simulink model "IK_corrado_old"  (R2023a)
settings: Solver=VariableStepAuto  StartTime=0.0  StopTime=15  MaxStep=0.05  RelTol=1e-2  AbsTol=1e-2  EnableMultiTasking=on
libraries: robotcorelib x1, robotmaniplib x1
settings Model: Creator=Savio Del Peschio  LastModifiedBy=Savio Del Peschio
settings SolverCC: AutoScaleAbsTol=off  AlgebraicLoopSolver=TrustRegion  MaxZcPerStep=1
settings DataIOCC: LimitDataPoints=on  MaxDataPoints=10000
settings OptimizationCC: ReuseModelBlockBuffer=off  LifeSpan=inf
settings DebuggingCC: UnconnectedInputMsg=warning  UnconnectedOutputMsg=warning  UnconnectedLineMsg=warning  AllowSymbolicDim=off  SFUnexpectedBacktrackingDiag=warning  SFNoUnconditionalDefaultTransitionDiag=warning  SFExecutionAtInitializationDiag=none  ArithmeticOperatorsInVariantConditions=warning
settings ModelReferenceCC: EnableRefExpFcnMdlSchedulingChecks=on
settings SFSimCC: SimUseLocalCustomCode=off  CustomCodeUndefinedFunction=UseInterfaceOnly
settings RTWCC: RTWUseLocalCustomCode=off  DLArmComputeVersion=19.05
settings CodeAppCC: StateflowObjectComments=on
settings GRTTargetCC: TargetLangStandard=C89/C90 (ANSI)
settings ConfigComp: CovMetricSettings=dw  CovSaveCumulativeToWorkspaceVar=on  CovSaveSingleToWorkspaceVar=on  CovExternalEMLEnable=off  CovSFcnEnable=off
settings SimscapeCC: SimscapeLogType=all  SimscapeLogSimulationStatistics=on  SimscapeLogDataHistory=10000

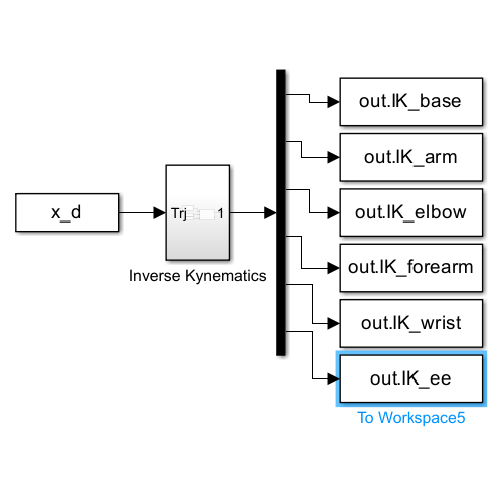
[thumbnail: Simulink's stored preview of the top-level diagram]
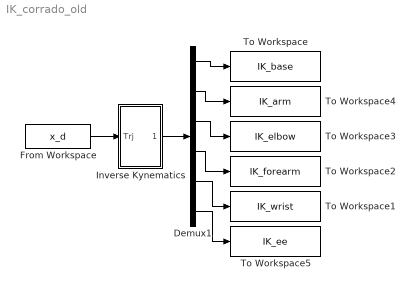
== system IK_corrado_old ==
  Demux1 : Demux  Outputs=6
  From Workspace : FromWorkspace  VariableName=x_d
  Inverse Kynematics : Subsystem
  To Workspace : ToWorkspace  VariableName=IK_base  SaveFormat=Timeseries  SampleTime=-1
  To Workspace1 : ToWorkspace  VariableName=IK_wrist  SaveFormat=Timeseries  SampleTime=-1
  To Workspace2 : ToWorkspace  VariableName=IK_forearm  SaveFormat=Timeseries  SampleTime=-1
  To Workspace3 : ToWorkspace  VariableName=IK_elbow  SaveFormat=Timeseries  SampleTime=-1
  To Workspace4 : ToWorkspace  VariableName=IK_arm  SaveFormat=Timeseries  SampleTime=-1
  To Workspace5 : ToWorkspace  VariableName=IK_ee  SaveFormat=Timeseries  SampleTime=-1
  wires:
  From Workspace/1 -> Inverse Kynematics/1(Trj)
  Demux1/1 -> To Workspace/1
  Demux1/4 -> To Workspace2/1
  Demux1/5 -> To Workspace1/1
  Demux1/2 -> To Workspace4/1
  Demux1/3 -> To Workspace3/1
  Inverse Kynematics/1(Outport) -> Demux1/1
  Demux1/6 -> To Workspace5/1

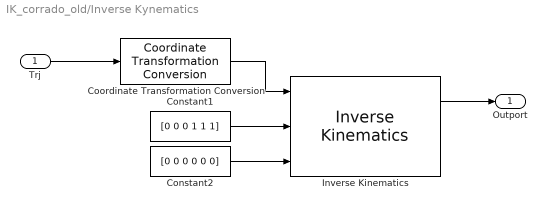
== system IK_corrado_old/Inverse Kynematics ==
  Trj : Inport
  Constant1 : Constant  Value=[0 0 0 1 1 1]
  Constant2 : Constant  Value=[0 0 0 0 0 0]
  Coordinate Transformation Conversion : robotcorelib/Coordinate Transformation Conversion  InputRepresentation=Translation Vector  InputEulerSequence=ZYX  ShowTrVecInputPort=on  OutputRepresentation=Homogeneous Transformation  OutputEulerSequence=ZYX  ShowTrVecOutputPort=on  SimulateUsing=Interpreted execution
  Inverse Kinematics : robotmaniplib/Inverse Kinematics  RigidBodyTree=corrado  EndEffector=Body6  ShowInfo=on  SolverName=BFGS Gradient Projection  EnforceJointLimits=on  MaxIterations=1500  MaxTime=10  GradientTolerance=1e-7  SolutionTolerance=1e-6  StepTolerance=1e-14  ErrorChangeTolerance=1e-12  UseErrorDamping=on  DampingBias=0.0025  SimulateUsing=Interpreted execution
  Outport : Outport
  wires:
  Constant2/1 -> Inverse Kinematics/3
  Constant1/1 -> Inverse Kinematics/2
  Coordinate Transformation Conversion/1 -> Inverse Kinematics/1
  Trj/1 -> Coordinate Transformation Conversion/1
  Inverse Kinematics/1 -> Outport/1
